simulink model "Adaptive_Control_2R_final"  (R2021a)
settings: Solver=ode4  StartTime=0.0  StopTime=2+dt  FixedStep=dt  RelTol=1e-3
settings Model: Creator=ravid  LastModifiedBy=Ashut
settings DebuggingCC: UnconnectedInputMsg=none  UnconnectedOutputMsg=none  UnconnectedLineMsg=none
settings RTWCC: DLArmComputeVersion=20.02.1

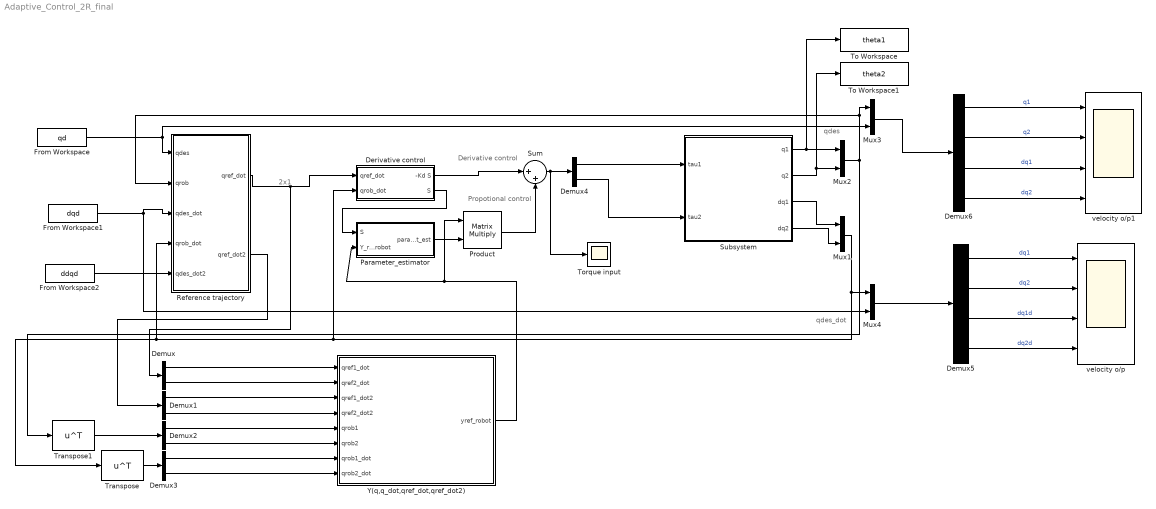
== system Adaptive_Control_2R_final ==
  note: qdes
  note: 2x1
  note: Derivative control
  note: qdes_dot
  note: Propotional control
  Demux{,1..4} (5 alike) : Demux  Outputs=2
  Demux5 : Demux
  Demux6 : Demux
  Derivative control : Subsystem
  From Workspace : FromWorkspace  VariableName=qd
  From Workspace1 : FromWorkspace  VariableName=dqd
  From Workspace2 : FromWorkspace  VariableName=ddqd
  Mux{1..4} (4 alike) : Mux  Inputs=2
  Parameter_estimator : Subsystem
  Product : Product  Multiplication=Matrix(*)  RndMeth=Zero
  Reference trajectory : Subsystem
  Subsystem : Subsystem
  Sum : Sum  Inputs=|++
  To Workspace : ToWorkspace  VariableName=theta1  SaveFormat=Timeseries  SampleTime=-1
  To Workspace1 : ToWorkspace  VariableName=theta2  SaveFormat=Timeseries  SampleTime=-1
  "Torque input " : Scope
  Transpose : Math  Operator=transpose  SaturateOnIntegerOverflow=on
  Transpose1 : Math  Operator=transpose  SaturateOnIntegerOverflow=on
  Y(q,q_dot,qref_dot,qref_dot2) : MATLAB Function  TreatAsAtomicUnit=on
  velocity o/p : Scope  NumInputPorts=4
  velocity o/p1 : Scope  NumInputPorts=4
  wires:
  From Workspace/1 -> Reference trajectory/1(qdes), Mux3/2
  Demux4/2 -> Subsystem/2(tau2)
  From Workspace1/1 -> Reference trajectory/3(qdes_dot), Mux4/2
  Parameter_estimator/1(paramt_est) -> Product/2
  Sum/1 -> "Torque input "/1, Demux4/1
  Mux2/1 -> Mux3/1, Reference trajectory/2(qrob), Transpose1/1
  From Workspace2/1 -> Reference trajectory/5(qdes_dot2)
  Demux2/1 -> Y(q,q_dot,qref_dot,qref_dot2)/5(qrob1)
  Demux4/1 -> Subsystem/1(tau1)
  Demux/1 -> Y(q,q_dot,qref_dot,qref_dot2)/1(qref1_dot)
  Reference trajectory/1(qref_dot) -> Derivative control/1(qref_dot), Demux/1
  Demux/2 -> Y(q,q_dot,qref_dot,qref_dot2)/2(qref2_dot)
  Derivative control/1(-Kd S) -> Sum/1
  Demux2/2 -> Y(q,q_dot,qref_dot,qref_dot2)/6(qrob2)
  Mux1/1 -> Transpose/1, Reference trajectory/4(qrob_dot), Derivative control/2(qrob_dot), Mux4/1
  Transpose/1 -> Demux3/1
  Reference trajectory/2(qref_dot2) -> Demux1/1
  Transpose1/1 -> Demux2/1
  Y(q,q_dot,qref_dot,qref_dot2)/1(yref_robot) -> Product/1, Parameter_estimator/2(Y_ref_robot)
  Derivative control/2(S) -> Parameter_estimator/1(S)
  Demux3/2 -> Y(q,q_dot,qref_dot,qref_dot2)/8(qrob2_dot)
  Demux1/1 -> Y(q,q_dot,qref_dot,qref_dot2)/3(qref1_dot2)
  Demux3/1 -> Y(q,q_dot,qref_dot,qref_dot2)/7(qrob1_dot)
  Demux1/2 -> Y(q,q_dot,qref_dot,qref_dot2)/4(qref2_dot2)
  Product/1 -> Sum/2
  Subsystem/1(q1) -> Mux2/1, To Workspace/1
  Subsystem/2(q2) -> To Workspace1/1, Mux2/2
  Subsystem/3(dq1) -> Mux1/1
  Subsystem/4(dq2) -> Mux1/2
  Mux4/1 -> Demux5/1
  Demux5/1 -> velocity o/p/1  "dq1"
  Demux5/2 -> velocity o/p/2  "dq2"
  Demux5/3 -> velocity o/p/3  "dq1d"
  Demux5/4 -> velocity o/p/4  "dq2d"
  Mux3/1 -> Demux6/1
  Demux6/1 -> velocity o/p1/1  "q1"
  Demux6/4 -> velocity o/p1/4  "dq2"
  Demux6/2 -> velocity o/p1/2  "q2"
  Demux6/3 -> velocity o/p1/3  "dq1"

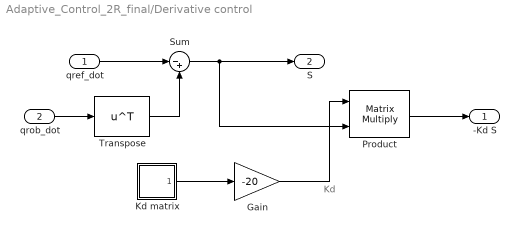
== system Adaptive_Control_2R_final/Derivative control ==
  note: Kd
  qref_dot : Inport
  qrob_dot : Inport  Port=2
  Gain : Gain  Gain=-20
  Kd matrix : Subsystem  Description=Replaced Block  mask(Replaced Block){}
      mask help: This block has been replaced with an empty subsystem because it used functionality that is unavailable in Simulink R2021a.
      mask Display: fprintf('Replaced: %s\n','IdentityMatrix')
  Product : Product  Multiplication=Matrix(*)  RndMeth=Zero
  Sum : Sum  Inputs=|-+
  Transpose : Math  Operator=transpose  SaturateOnIntegerOverflow=on
  -Kd S : Outport
  S : Outport  Port=2
  wires:
  qref_dot/1 -> Sum/1
  Sum/1 -> S/1, Product/2
  Kd matrix/1(Out1) -> Gain/1
  Product/1 -> -Kd S/1
  qrob_dot/1 -> Transpose/1
  Transpose/1 -> Sum/2
  Gain/1 -> Product/1

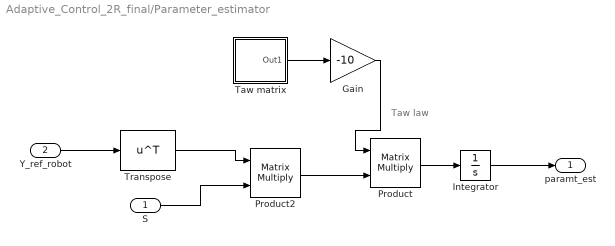
== system Adaptive_Control_2R_final/Parameter_estimator ==
  note: Taw law
  S : Inport
  Y_ref_robot : Inport  Port=2
  Gain : Gain  Gain=-10
  Integrator : Integrator
  Product : Product  Multiplication=Matrix(*)  RndMeth=Zero
  Product2 : Product  Multiplication=Matrix(*)  RndMeth=Zero
  Taw matrix : Subsystem  Description=Replaced Block  mask(Replaced Block){}
      mask help: This block has been replaced with an empty subsystem because it used functionality that is unavailable in Simulink R2021a.
      mask Display: fprintf('Replaced: %s\n','IdentityMatrix')
  Transpose : Math  Operator=transpose  SaturateOnIntegerOverflow=on
  paramt_est : Outport
  wires:
  Product/1 -> Integrator/1
  Integrator/1 -> paramt_est/1
  Taw matrix/1(Out1) -> Gain/1
  Gain/1 -> Product/1
  Product2/1 -> Product/2
  Y_ref_robot/1 -> Transpose/1
  Transpose/1 -> Product2/1
  S/1 -> Product2/2

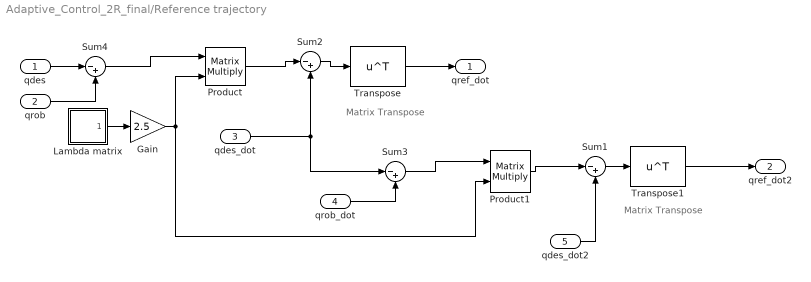
== system Adaptive_Control_2R_final/Reference trajectory ==
  note: Matrix Transpose
  note: Matrix Transpose
  qdes : Inport
  qrob : Inport  Port=2
  qdes_dot : Inport  Port=3
  qrob_dot : Inport  Port=4
  qdes_dot2 : Inport  Port=5
  Gain : Gain  Gain=2.5
  Lambda matrix : Subsystem  Description=Replaced Block  mask(Replaced Block){}
      mask help: This block has been replaced with an empty subsystem because it used functionality that is unavailable in Simulink R2021a.
      mask Display: fprintf('Replaced: %s\n','IdentityMatrix')
  Product : Product  Multiplication=Matrix(*)  RndMeth=Zero
  Product1 : Product  Multiplication=Matrix(*)  RndMeth=Zero
  Sum{1..4} (4 alike) : Sum  Inputs=|-+
  Transpose : Math  Operator=transpose  SaturateOnIntegerOverflow=on
  Transpose1 : Math  Operator=transpose  SaturateOnIntegerOverflow=on
  qref_dot : Outport
  qref_dot2 : Outport  Port=2
  wires:
  qdes/1 -> Sum4/1
  qrob/1 -> Sum4/2
  Sum4/1 -> Product/1
  Lambda matrix/1(Out1) -> Gain/1
  Gain/1 -> Product/2, Product1/2
  Product/1 -> Sum2/1
  qdes_dot/1 -> Sum2/2, Sum3/1
  qrob_dot/1 -> Sum3/2
  Sum3/1 -> Product1/1
  Product1/1 -> Sum1/1
  qdes_dot2/1 -> Sum1/2
  Transpose/1 -> qref_dot/1
  Sum2/1 -> Transpose/1
  Sum1/1 -> Transpose1/1
  Transpose1/1 -> qref_dot2/1

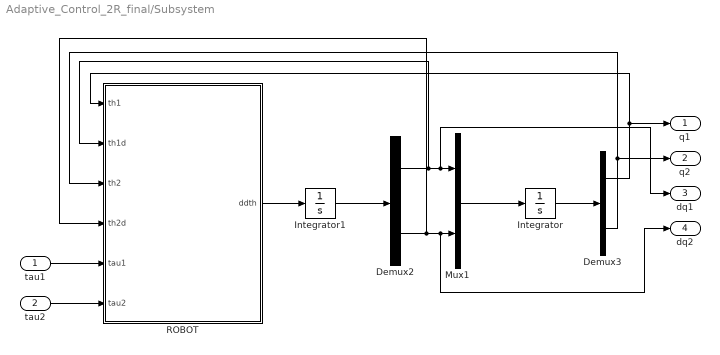
== system Adaptive_Control_2R_final/Subsystem ==
  tau1 : Inport
  tau2 : Inport  Port=2
  Demux2 : Demux  Outputs=2
  Demux3 : Demux  Outputs=2
  Integrator : Integrator  InitialCondition=[0;pi/2]
  Integrator1 : Integrator  InitialCondition=[0;0]
  Mux1 : Mux  Inputs=2
  ROBOT : MATLAB Function  TreatAsAtomicUnit=on
  q1 : Outport
  q2 : Outport  Port=2
  dq1 : Outport  Port=3
  dq2 : Outport  Port=4
  wires:
  Demux2/1 -> ROBOT/2(th1d), dq1/1, Mux1/1
  ROBOT/1(ddth) -> Integrator1/1
  Integrator/1 -> Demux3/1
  Demux3/1 -> q1/1, ROBOT/1(th1)
  Mux1/1 -> Integrator/1
  Demux2/2 -> ROBOT/4(th2d), dq2/1, Mux1/2
  Demux3/2 -> q2/1, ROBOT/3(th2)
  Integrator1/1 -> Demux2/1
  tau1/1 -> ROBOT/5(tau1)
  tau2/1 -> ROBOT/6(tau2)

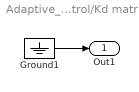
== system Adaptive_Control_2R_final/Derivative control/Kd matrix ==
  Ground1 : Ground
  Out1 : Outport
  wires:
  Ground1/1 -> Out1/1

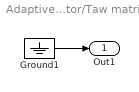
== system Adaptive_Control_2R_final/Parameter_estimator/Taw matrix ==
  Ground1 : Ground
  Out1 : Outport
  wires:
  Ground1/1 -> Out1/1

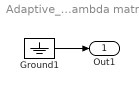
== system Adaptive_Control_2R_final/Reference trajectory/Lambda matrix ==
  Ground1 : Ground
  Out1 : Outport
  wires:
  Ground1/1 -> Out1/1

== matlab function Adaptive_Control_2R_final/Y(q,q_dot,qref_dot,qref_dot2) ==
  data: qref1_dot input; yref_robot output; qref2_dot input; qref1_dot2 input; qref2_dot2 input; qrob1 input; qrob2 input; qrob1_dot input; qrob2_dot input
function yref_robot = fcn(qref1_dot,qref2_dot,qref1_dot2,qref2_dot2,qrob1,qrob2,qrob1_dot,qrob2_dot)
%#eml

yref_robot = [qref1_dot2+qref2_dot2, ( cos(qrob2)*(2*qref1_dot2 + qref2_dot2))-((sin(qrob2))*((qref1_dot*qrob2_dot)+(qref2_dot*qrob1_dot)+(qref2_dot*qrob2_dot))),qref1_dot2, 9.8* cos(qrob1), (9.8 * cos(qrob1+qrob2)) ;
    qref1_dot2+qref2_dot2, ((qref1_dot2 * cos(qrob2))+ (qrob1_dot * qref1_dot * sin(qrob2))), 0,0, cos(qrob1+qrob2)];

== matlab function Adaptive_Control_2R_final/Subsystem/ROBOT ==
  data: th1 input; ddth output; th1d input; th2 input; th2d input; tau1 input; tau2 input
function ddth= ode_solver_script_q1_a(th1,th1d,th2,th2d,tau1,tau2)
x = [th1;th1d;th2;th2d];
%% Input parameters
m2=1; m1=1; l1=1; l2=1; g=9.81;


%% Equation of motion 

%M matrix
M11=((((m1/3) + m2)*l1^2) +((m2/3)*l2^2) + (m2*l1*l2*cos(x(3))));
M12=(m2*(((l2^2)/3) + (0.5*l1*l2*cos(x(3)))));
M21=M12;
M22=((1/3)*m2*l2*l2);

%H matrix
H1 =((-m2*l1*l2*sin(x(3))*x(2)*x(4)) - (0.5*m2*l1*l2*sin(x(3))*x(4)*x(4)));
H2 = (0.5 * m2* l1*l2*sin(x(3))*x(2)*x(2));

%G matrix
G1=( ((((0.5*m1) + m2)*l1*cos(x(1))) + (0.5*m2*l2*cos(x(1)+x(3))))*g);
G2=0.5*m2*l2*cos(x(1)+x(3))*g;



M=[M11 M12;M21 M22];

HG = [H1 + G1; H2 + G2];

T=[tau1; tau2];

%% Equation in terms of acceleration

ddth = (inv(M)) * (T - HG)    ;% Joint  accelaration
